simulink model "plant_model"  (R2026a)
settings: Solver=ode4  FixedStep=0.001
undefined symbols (not defined in the file): J_wheel, K_brake, m_vehicle, R_wheel, ROAD_TYPE, v0
settings Model: Creator=anh  LastModifiedBy=anh

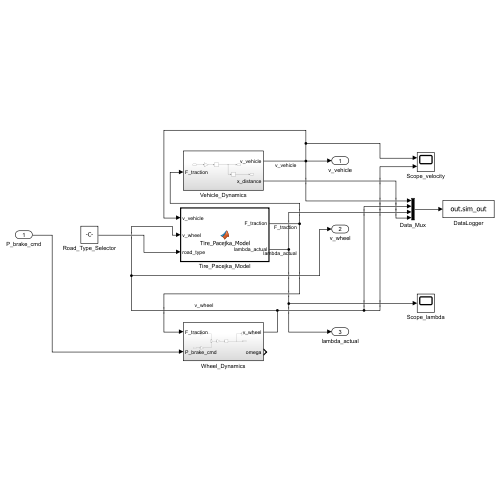
[thumbnail: Simulink's stored preview of the top-level diagram]
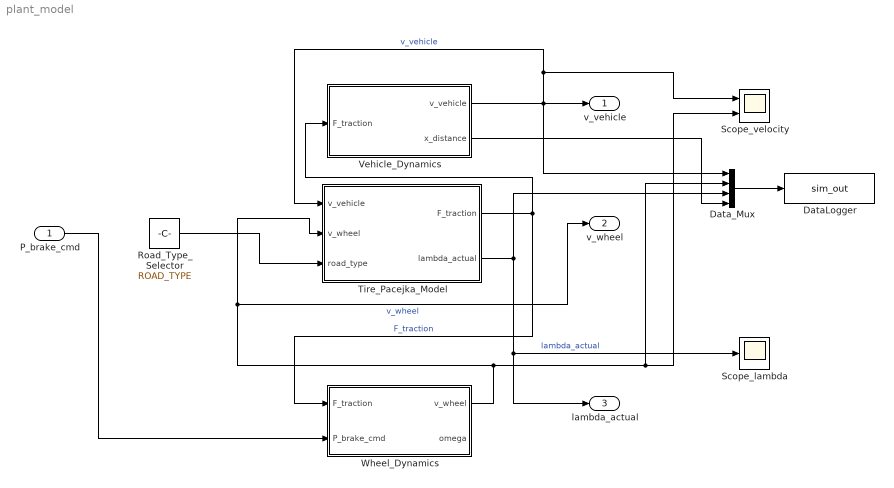
== system plant_model ==
  P_brake_cmd : Inport
  DataLogger : ToWorkspace  VariableName=sim_out  SaveFormat=Structure With Time  SampleTime=-1
  Data_Mux : Mux
  Road_Type_Selector : Constant  Value=ROAD_TYPE
  Scope_lambda : Scope
      settings: ActiveDisplayYMinimum=-0.12499999999999997  ActiveDisplayYMaximum=1.125
  Scope_velocity : Scope  NumInputPorts=2
      settings: ActiveDisplayYMinimum=-3.4722222222222214  ActiveDisplayYMaximum=31.25
  Tire_Pacejka_Model : MATLAB Function  TreatAsAtomicUnit=on
  Vehicle_Dynamics : Subsystem
  Wheel_Dynamics : Subsystem
  v_vehicle : Outport
  v_wheel : Outport  Port=2
  lambda_actual : Outport  Port=3
  wires:
  Road_Type_Selector/1 -> Tire_Pacejka_Model/3(road_type)
  Tire_Pacejka_Model/1(F_traction) -> Vehicle_Dynamics/1(F_traction), Wheel_Dynamics/1(F_traction)  "F_traction"
  Vehicle_Dynamics/1(v_vehicle) -> Tire_Pacejka_Model/1(v_vehicle), Scope_velocity/1, v_vehicle/1, Data_Mux/1  "v_vehicle"
  Wheel_Dynamics/1(v_wheel) -> Data_Mux/2, Scope_velocity/2, v_wheel/1, Tire_Pacejka_Model/2(v_wheel)  "v_wheel"
  Tire_Pacejka_Model/2(lambda_actual) -> Scope_lambda/1, lambda_actual/1, Data_Mux/3  "lambda_actual"
  Vehicle_Dynamics/2(x_distance) -> Data_Mux/4
  Data_Mux/1 -> DataLogger/1
  P_brake_cmd/1 -> Wheel_Dynamics/2(P_brake_cmd)

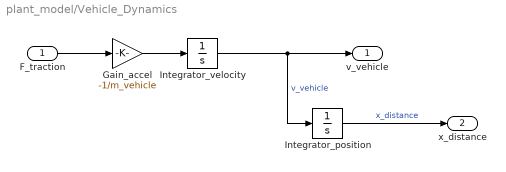
== system plant_model/Vehicle_Dynamics ==
  F_traction : Inport
  Gain_accel : Gain  Gain=-1/m_vehicle
  Integrator_position : Integrator
  Integrator_velocity : Integrator  InitialCondition=v0  LimitOutput=on  LowerSaturationLimit=0
  v_vehicle : Outport
  x_distance : Outport  Port=2
  wires:
  F_traction/1 -> Gain_accel/1
  Gain_accel/1 -> Integrator_velocity/1
  Integrator_velocity/1 -> v_vehicle/1, Integrator_position/1  "v_vehicle"
  Integrator_position/1 -> x_distance/1  "x_distance"

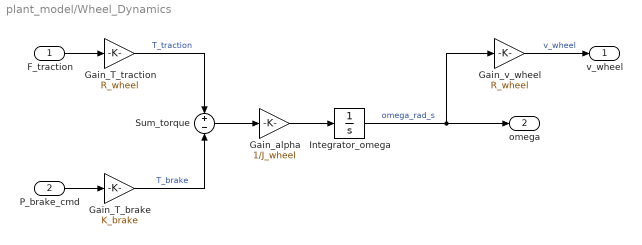
== system plant_model/Wheel_Dynamics ==
  F_traction : Inport
  P_brake_cmd : Inport  Port=2
  Gain_T_brake : Gain  Gain=K_brake
  Gain_T_traction : Gain  Gain=R_wheel
  Gain_alpha : Gain  Gain=1/J_wheel
  Gain_v_wheel : Gain  Gain=R_wheel
  Integrator_omega : Integrator  InitialCondition=v0 / R_wheel  LimitOutput=on  LowerSaturationLimit=0
  Sum_torque : Sum  Inputs=+-
  v_wheel : Outport
  omega : Outport  Port=2
  wires:
  F_traction/1 -> Gain_T_traction/1
  P_brake_cmd/1 -> Gain_T_brake/1
  Gain_T_traction/1 -> Sum_torque/1  "T_traction"
  Gain_T_brake/1 -> Sum_torque/2  "T_brake"
  Sum_torque/1 -> Gain_alpha/1
  Gain_alpha/1 -> Integrator_omega/1
  Integrator_omega/1 -> omega/1, Gain_v_wheel/1  "omega_rad_s"
  Gain_v_wheel/1 -> v_wheel/1  "v_wheel"

== matlab function plant_model/Tire_Pacejka_Model ==
  data: v_vehicle input; F_traction output; v_wheel input; road_type input; lambda_actual output
function [F_traction, lambda_actual] = Tire_Pacejka_Model(v_vehicle, v_wheel, road_type)
%TIRE_PACEJKA_MODEL  Tinh luc keo (F_traction) va slip ratio thuc te (lambda_actual).
%
%  Inputs:
%    v_vehicle   - Van toc xe (than xe) [m/s]
%    v_wheel     - Van toc tuyen tinh banh xe [m/s]
%    road_type   - Loai mat duong: 1=Kho, 2=Uot, 3=Da soi
%
%  Outputs:
%    F_traction  - Luc keo tu lop [N]  (can chuyen dong)
%    lambda_actual - Slip ratio thuc te [-], pham vi [0, 1]
%
%  Thong so vat ly khop voi init_params.m:
%    m_vehicle = 612.5 kg (khoi luong 1/4 xe Ford Everest)
%    g         = 9.81 m/s2

%% Thong so vat ly (hardcode de tuong thich voi code generation)
m_veh = 612.5;   % [kg]
g     = 9.81;    % [m/s2]

%% Tinh slip ratio (co bao ve chia cho 0)
if v_vehicle < 0.1
    % Xe da dung hoac gan dung: khong co slip co nghia
    lambda_actual = 0.0;
else
    lambda_actual = (v_vehicle - v_wheel) / v_vehicle;
end

% Clamp vao pham vi vat ly [0, 1]
lambda_actual = max(0.0, min(1.0, lambda_actual));

%% Chon tham so Pacejka theo loai mat duong
switch road_type
    case 1   % Nhua kho (Dry Asphalt)
        B = 10.0;  C = 1.90;  D = 0.90;  E = 0.97;
    case 2   % Nhua uot (Wet Asphalt)
        B = 8.0;   C = 1.70;  D = 0.50;  E = 0.80;
    case 3   % Da soi / Bang tuyet (Gravel / Ice)
        B = 6.0;   C = 1.50;  D = 0.30;  E = 0.60;
    otherwise
        % Default: nhua kho
        B = 10.0;  C = 1.90;  D = 0.90;  E = 0.97;
end

%% Pacejka Magic Formula
% mu(lambda) = D * sin(C * atan(B*lambda - E*(B*lambda - atan(B*lambda))))
phi = B * lambda_actual;
mu  = D * sin(C * atan(phi - E * (phi - atan(phi))));
mu  = max(0.0, mu);   % He so ma sat khong the am

%% Luc keo tu lop len mat duong
F_traction = mu * m_veh * g;   % [N]

end
